simulink model "initial_simulation_inverse"  (R2018b)
settings: Solver=VariableStepAuto  StartTime=0.0  StopTime=10.0  RelTol=1e-3
settings Model: Creator=299792458  LastModifiedBy=299792458

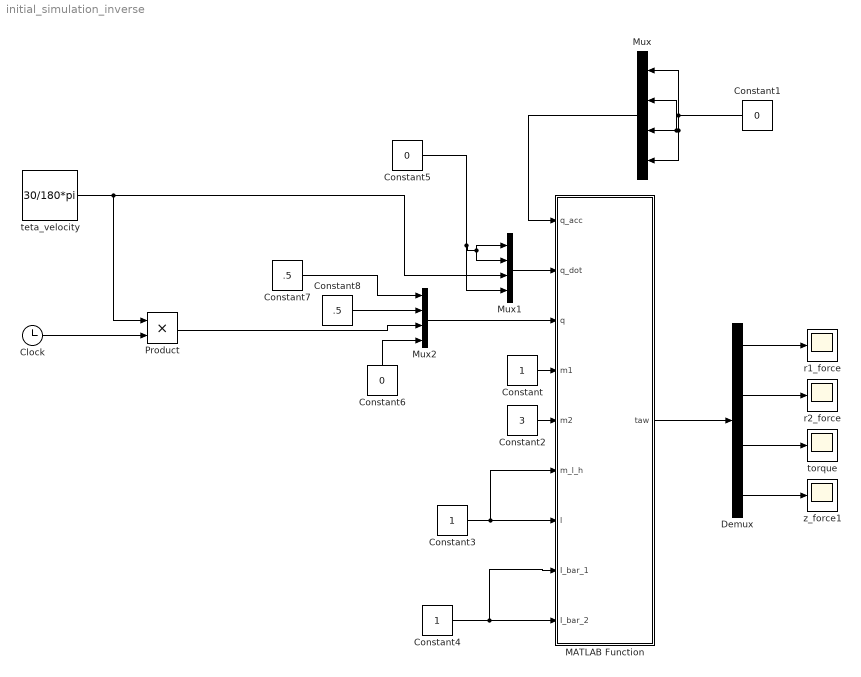
== system initial_simulation_inverse ==
  Clock : Clock
  Constant : Constant
  Constant1 : Constant  Value=0
  Constant2 : Constant  Value=3
  Constant3 : Constant
  Constant4 : Constant
  Constant5 : Constant  Value=0
  Constant6 : Constant  Value=0
  Constant7 : Constant  Value=.5
  Constant8 : Constant  Value=.5
  Demux : Demux
  MATLAB Function : MATLAB Function  TreatAsAtomicUnit=on
  Mux : Mux
  Mux1 : Mux
  Mux2 : Mux
  Product : Product
  r1_force : Scope
  r2_force : Scope
  teta_velocity : Constant  Value=30/180*pi
  torque : Scope
  z_force1 : Scope
  wires:
  Constant6/1 -> Mux2/4
  Demux/1 -> r1_force/1
  Demux/4 -> z_force1/1
  Constant4/1 -> MATLAB Function/9(I_bar_2), MATLAB Function/8(I_bar_1)
  Constant5/1 -> Mux1/4, Mux1/2, Mux1/1
  Demux/3 -> torque/1
  Constant/1 -> MATLAB Function/4(m1)
  MATLAB Function/1(taw) -> Demux/1
  Mux/1 -> MATLAB Function/1(q_acc)
  Demux/2 -> r2_force/1
  Constant1/1 -> Mux/3, Mux/2, Mux/4, Mux/1
  Constant3/1 -> MATLAB Function/6(m_l_h), MATLAB Function/7(l)
  teta_velocity/1 -> Product/1, Mux1/3
  Constant7/1 -> Mux2/1
  Mux1/1 -> MATLAB Function/2(q_dot)
  Product/1 -> Mux2/3
  Constant2/1 -> MATLAB Function/5(m2)
  Mux2/1 -> MATLAB Function/3(q)
  Constant8/1 -> Mux2/2
  Clock/1 -> Product/2

== matlab function initial_simulation_inverse/MATLAB Function ==
  data: q_acc input; q_dot input; q input; m1 input; taw output; m2 input; m_l_h input; l input; I_bar_1 input; I_bar_2 input
function taw = fcn(q_acc,q_dot, q,m1,m2,m_l_h,l,I_bar_1,I_bar_2)
% q=[r1;r2;theta;z];
% q_dot=[r1_d;r2_d;theta_d;z_d];
g=9.80665;
M_mat =[ m1,0,0,0
    0, m2,0,0
    0,  0, (7*m_l_h*l^2)/27 + m1*q(1,1)^2 + m2*q(2,1)^2 + I_bar_1 + I_bar_2 ,               0
    0,  0,0, m1 + m2 + m_l_h];

G_vec=[0
    0
    0
    g*(m1 + m2 + m_l_h)];

C_mat=[0,0,-m1*q(1,1)*q_dot(3,1), 0
    0,0, -m2*q(2,1)*q_dot(3,1), 0
    2*m1*q(1,1)*q_dot(3,1), 2*m2*q(2,1)*q_dot(3,1), 0, 0
    0,0, 0, 0];


taw=M_mat*q_acc+C_mat*q_dot+G_vec;
end
